simulink model "MaxonStateSpace"  (R2018a)
settings: Solver=VariableStepAuto  StartTime=0.0  StopTime=10  RelTol=1e-3
libraries: simulink x1
settings Model: Creator=pei-T  LastModifiedBy=pei-T

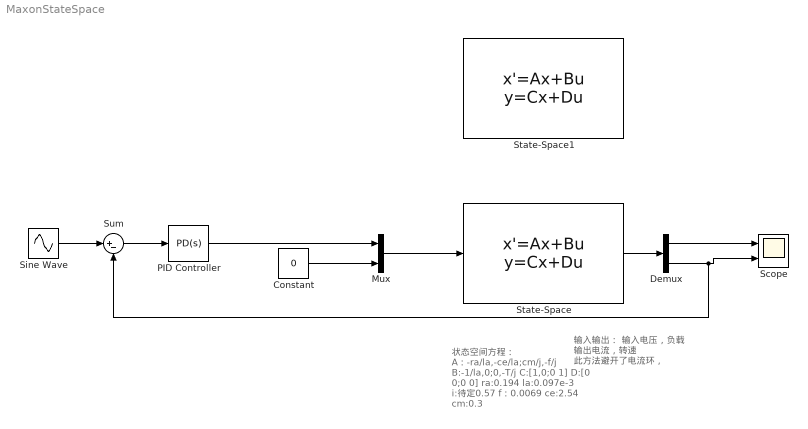
== system MaxonStateSpace ==
  note: 输入输出：
      | 输入电压，负载
      | 输出电流，转速
      | 此方法避开了电流环，
  note: 状态空间方程：
      |
      |
      | A：-ra/la,-ce/la;cm/j,-f/j
      | B:-1/la,0;0,-T/j
      | C:[1,0;0 1]
      | D:[0 0;0 0]
      | ra:0.194
      | la:0.097e-3
      | i:待定0.57
      | f：0.0069
      | ce:2.54
      | cm:0.3
  Constant : Constant  Value=0
  Demux : Demux  Outputs=2
  Mux : Mux  Inputs=2
  PID Controller : simulink/Continuous/PID Controller  Controller=PD  TimeDomain=Continuous-time  SampleTime=-1  IntegratorMethod=Forward Euler  FilterMethod=Forward Euler  Form=Parallel  UseFilter=on  ControllerParametersSource=internal  P=-187.503942894087  I=1  D=0  N=100  InitialConditionSource=internal  InitialConditionForIntegrator=0  InitialConditionForFilter=0  ExternalReset=none  LimitOutput=on  UpperSaturationLimit=24  LowerSaturationLimit=-24  LinearizeAsGain=on  AntiWindupMode=none  Kb=1  TrackingMode=off  Kt=1  PParamMin=[]  PParamMax=[]  IParamMin=[]  IParamMax=[]  DParamMin=[]  DParamMax=[]  NParamMin=[]  NParamMax=[]  KbParamMin=[]  KbParamMax=[]  KtParamMin=[]  KtParamMax=[]  POutMin=[]  POutMax=[]  IOutMin=[]  IOutMax=[]  DOutMin=[]  DOutMax=[]  NOutMin=[]  NOutMax=[]  KbOutMin=[]  KbOutMax=[]  KtOutMin=[]  KtOutMax=[]  IntegratorOutMin=[]  IntegratorOutMax=[]  FilterOutMin=[]  FilterOutMax=[]  SumOutMin=[]  SumOutMax=[]  SumI1OutMin=[]  SumI1OutMax=[]  SumI2OutMin=[]  SumI2OutMax=[]  SumI3OutMin=[]  SumI3OutMax=[]  SumDOutMin=[]  SumDOutMax=[]  SaturationOutMin=[]  SaturationOutMax=[]  IntegratorContinuousStateAttributes=''  IntegratorStateMustResolveToSignalObject=off  IntegratorRTWStateStorageClass=Auto  FilterContinuousStateAttributes=''  FilterStateMustResolveToSignalObject=off  FilterRTWStateStorageClass=Auto  DifferentiatorICPrevScaledInput=0  DifferentiatorOutMin=[]  DifferentiatorOutMax=[]  FilterDiffOutCoefMin=[]  FilterDiffOutCoefMax=[]  SumDenOutMin=[]  SumDenOutMax=[]  SumNumOutMin=[]  SumNumOutMax=[]  ReciprocalOutMin=[]  ReciprocalOutMax=[]  DivideOutMin=[]  DivideOutMax=[]  TunerSelectOption=Transfer Function Based (PID Tuner App)
  Scope : Scope  NumInputPorts=2
  Sine Wave : Sin  Amplitude=1000  SampleTime=0
  State-Space : StateSpace  A=[-2000 -26185;0.52, -0.00121]  B=[-1030900 0;0 -1.7544]  C=[1,0;0 1]  D=[0 0;0 0]  InitialCondition=0
  State-Space1 : StateSpace  A=[-2000 -26185;0.52, -0.00121]  B=[-10309 0;0 -1.7544]  C=[1,0;0 1]  D=[0 0;0 0]  InitialCondition=0
  Sum : Sum  Inputs=|+-
  wires:
  Mux/1 -> State-Space/1
  Constant/1 -> Mux/2
  PID Controller/1 -> Mux/1
  State-Space/1 -> Demux/1
  Demux/1 -> Scope/1
  Demux/2 -> Sum/2, Scope/2
  Sum/1 -> PID Controller/1
  Sine Wave/1 -> Sum/1
